simulink model "LQG_model"  (R2018b)
settings: Solver=FixedStepDiscrete  StartTime=0.0  StopTime=1.5  FixedStep=Ts  RelTol=1e-3
values from neighbouring files (symbols this model uses):
  Ad = expm(Av*Ts)    [main.m]
  Bd = double(int(exp_At,t,0,Ts)*Bv)    [main.m]
  C1v = repl(C1)    [main.m]
  K_fb = Klqr(:,1:length(Ad))    [main.m]
  K_I = Klqr(:,length(Ad)+1:end)*20    [main.m]
  sigma2_phi2 = calcVariance(0.02, 0.997)    [main.m]
  sigma2_Te = calcVariance(0.1, 0.997)    [main.m]
  sigma2_va = calcVariance(0.3, 0.997)    [main.m]
  sigma2_w2 = calcVariance(0.01, 0.997)    [main.m]
  Ts = 1e-3    (= 0.001)    [main.m]
  x0 = [0 0 0 0 0]'    [main.m]
undefined symbols (not defined in the file or in its folder): DiscIntNeverNeededParam, L_kalman, sigbuilder_block
settings Model: Creator=Renata  LastModifiedBy=Renata

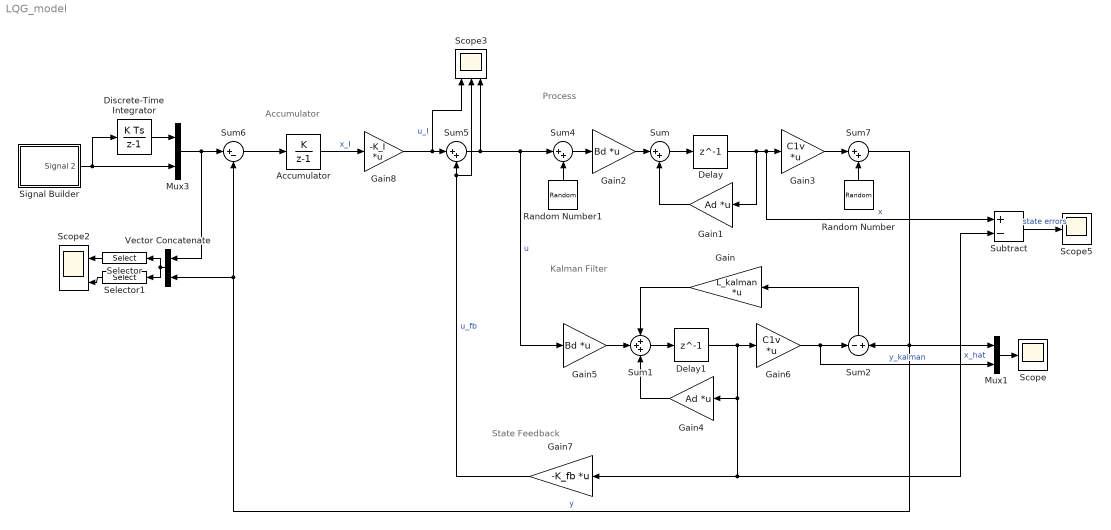
== system LQG_model ==
  note: State Feedback
  note: Accumulator
  note: Kalman Filter
  note: Process
  Accumulator : DiscreteIntegrator  IntegratorMethod=Accumulation: Forward Euler  SampleTime=-1  ICPrevOutput=DiscIntNeverNeededParam  ICPrevScaledInput=DiscIntNeverNeededParam
  Delay : Delay  DelayLength=1  InitialCondition=x0
  Delay1 : Delay  DelayLength=1
  Discrete-Time Integrator : DiscreteIntegrator  SampleTime=-1  ICPrevOutput=DiscIntNeverNeededParam  ICPrevScaledInput=DiscIntNeverNeededParam
  Gain : Gain  Gain=L_kalman  Multiplication=Matrix(K*u)
  Gain1 : Gain  Gain=Ad  Multiplication=Matrix(K*u)
  Gain2 : Gain  Gain=Bd  Multiplication=Matrix(K*u)
  Gain3 : Gain  Gain=C1v  Multiplication=Matrix(K*u)
  Gain4 : Gain  Gain=Ad  Multiplication=Matrix(K*u)
  Gain5 : Gain  Gain=Bd  Multiplication=Matrix(K*u)
  Gain6 : Gain  Gain=C1v  Multiplication=Matrix(K*u)
  Gain7 : Gain  Gain=-K_fb  Multiplication=Matrix(K*u)
  Gain8 : Gain  Gain=-K_I  Multiplication=Matrix(K*u)
  Mux1 : Mux  Inputs=2
  Mux3 : Mux  Inputs=2
  Random Number : RandomNumber  Variance=[sigma2_phi2 sigma2_w2]  SampleTime=Ts
  Random Number1 : RandomNumber  Variance=[sigma2_va,sigma2_Te]  SampleTime=Ts
  Scope : Scope
  Scope2 : Scope  NumInputPorts=2
  Scope3 : Scope  NumInputPorts=3
  Scope5 : Scope
  Selector : Selector  InputPortWidth=4  IndexOptions=Index vector (dialog)  Indices=[1 3]  OutputSizes=1
  Selector1 : Selector  InputPortWidth=4  IndexOptions=Index vector (dialog)  Indices=[2 4]  OutputSizes=1
  Signal Builder : Subsystem  Tag=STV Subsys  LoadFcn=sigbuilder_block('load');  StartFcn=sigbuilder_block('start');  StopFcn=sigbuilder_block('stop');  ClipboardFcn=sigbuilder_block('clipboard');  mask(Sigbuilder block){tuvar=[0:10]}
      mask help: Simulink:masks:SigbuilderBlock_MD
      mask init:
      | if ~strcmp(get_param(bdroot(gcbh),'SimulationStatus'),'stopped') tuvar = sigbuilder_block('maskInit'); end
      settings: CopyFcn=sigbuilder_block('copy');  DeleteFcn=sigbuilder_block('delete');  ModelCloseFcn=sigbuilder_block('modelClose');  PreSaveFcn=sigbuilder_block('preSave');  PauseFcn=sigbuilder_block('pause');  ContinueFcn=sigbuilder_block('continue');  NameChangeFcn=sigbuilder_block('namechange');  OpenFcn=sigbuilder_block('open',[367.8 74.4 682.2 467.4 ]);  CloseFcn=sigbuilder_block('close');
      mask Display: plot(0, 0, 100, 100,[2, 2, 32, 32, 2], [68, 8, 8, 68, 68],[32, 2], [38, 38], [32, 19, 2],[53, 60, 44], [32, 17, 17, 2],[16, 16, 31, 31]);txt = getActiveGroup(gcbh);text(2, 100, txt,'verticalAlignment', 'top');
  Subtract : Sum  Inputs=+-
  Sum{,4..5,7} (4 alike) : Sum  Inputs=|++
  Sum1 : Sum  Inputs=+++
  Sum2 : Sum  Inputs=-|+
  Sum6 : Sum  Inputs=|+-
  Vector Concatenate : Concatenate
  wires:
  Delay/1 -> Subtract/1, Gain3/1, Gain1/1  "x"
  Sum/1 -> Delay/1
  Gain1/1 -> Sum/2
  Gain2/1 -> Sum/1
  Gain5/1 -> Sum1/2
  Delay1/1 -> Gain6/1, Gain7/1, Subtract/2, Gain4/1  "x_hat"
  Gain4/1 -> Sum1/3
  Sum1/1 -> Delay1/1
  Gain6/1 -> Mux1/2, Sum2/1  "y_kalman"
  Sum7/1 -> Sum2/2, Mux1/1, Sum6/2, Vector Concatenate/2  "y"
  Gain3/1 -> Sum7/1
  Sum4/1 -> Gain2/1
  Gain7/1 -> Scope3/2, Sum5/2  "u_fb"
  Sum2/1 -> Gain/1
  Gain/1 -> Sum1/1
  Sum5/1 -> Sum4/1, Gain5/1, Scope3/3  "u"
  Random Number/1 -> Sum7/2
  Random Number1/1 -> Sum4/2
  Gain8/1 -> Sum5/1, Scope3/1  "u_I"
  Sum6/1 -> Accumulator/1
  Accumulator/1 -> Gain8/1  "x_I"
  Mux1/1 -> Scope/1
  Subtract/1 -> Scope5/1  "state errors"
  Mux3/1 -> Vector Concatenate/1, Sum6/1
  Signal Builder/1(Signal 2) -> Discrete-Time Integrator/1, Mux3/2
  Discrete-Time Integrator/1 -> Mux3/1
  Selector/1 -> Scope2/1
  Vector Concatenate/1 -> Selector/1, Selector1/1
  Selector1/1 -> Scope2/2

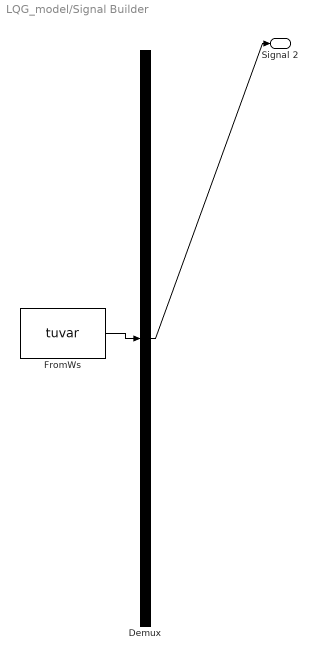
== system LQG_model/Signal Builder ==
  Demux : Demux  Tag=STV Demux  Outputs=1
  FromWs : FromWorkspace  Tag=STV FromWs  VariableName=tuvar  SampleTime=0
      SigBuilderData=|
      | common.afterFinalStr = 'Extrapolate'
      | common.sampleTime = 0
      | dataSet.timeRange = [0 10]
      | dataSet.name = 'Group 1'
      | sbobj.Groups.Name = 'Group 1'
      | sbobj.Groups.Signals.Name = 'Signal 2'
      | sbobj.Groups.Signals.XData = [0 0.5 0.5 10]
      | sbobj.Groups.Signals.YData = [10 10 100 100]
  Signal 2 : Outport  Tag=STV Outport
  wires:
  FromWs/1 -> Demux/1
  Demux/1 -> Signal 2/1
